simulink model "RPBSIDblocks"  (Simulink 7.4)
settings: Solver=ode45  StartTime=0.0  StopTime=10.0  RelTol=1e-3
undefined symbols (not defined in the file): Du, Dy, W
libraries: cstblocks x1
(part 1 of 2)
settings Model: Creator=ivohoutzager  LastModifiedBy=Ivo
settings OptimizationCC: InitFltsAndDblsToZero=on
settings DebuggingCC: SaveWithParameterizedLinksMsg=none  MultiTaskCondExecSysMsg=none
settings HardwareCC: TargetHWDeviceType=32-bit Generic
settings RTWCC: IncludeERTFirstTime=on
settings GRTTargetCC: TargetFcnLib=ansi_tfl_tmw.mat

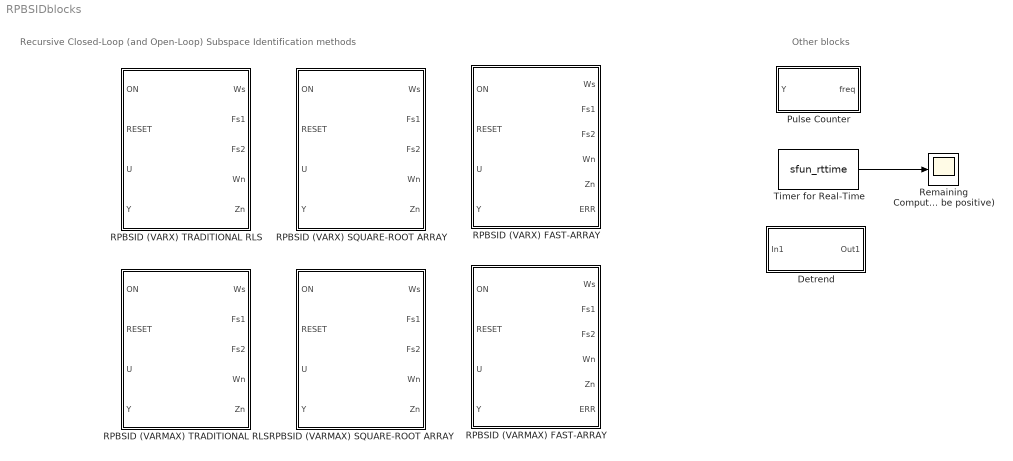
== system RPBSIDblocks ==
  note: Recursive Closed-Loop (and Open-Loop)
      | Subspace Identification methods
  note: Other blocks
  Detrend : Subsystem
  Pulse Counter : Stateflow chart
  RPBSID (VARMAX) FAST-ARRAY : Stateflow chart
  RPBSID (VARMAX) SQUARE-ROOT ARRAY : Stateflow chart
  RPBSID (VARMAX) TRADITIONAL RLS : Stateflow chart
  RPBSID (VARX) FAST-ARRAY : Stateflow chart
  RPBSID (VARX) SQUARE-ROOT ARRAY : Stateflow chart
  RPBSID (VARX) TRADITIONAL RLS : Stateflow chart
  Remaining Computation Time (must be positive) : Scope
      settings: TimeRange=10  YMin=-0.01  YMax=0.01
  Timer for Real-Time : S-Function  FunctionName=sfun_rttime  Parameters=1  EnableBusSupport=off
  wires:
  Timer for Real-Time/1 -> Remaining Computation Time (must be positive)/1

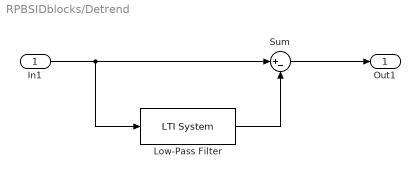
== system RPBSIDblocks/Detrend ==
  In1 : Inport  OutDataType=fixdt(1, 16)  OutScaling=2^0
  Low-Pass Filter : cstblocks/LTI System  SystemSampleTime=-1  sys=LP  IC=[]
  Sum : Sum  Inputs=|+-  OutDataType=fixdt(1, 16)  OutScaling=2^0
  Out1 : Outport  OutDataType=fixdt(1, 16)  OutScaling=2^0
  wires:
  In1/1 -> Low-Pass Filter/1, Sum/1
  Low-Pass Filter/1 -> Sum/2
  Sum/1 -> Out1/1

== matlab function RPBSID (VARMAX) SQUARE-ROOT ARRAY ==
  data: ON input double; RESET input double; Ws output double; Fs1 output double; Fs2 output double; U input double; Y input double size=2; Wn output double; Zn output double; W parameter double; Du parameter double; Dy parameter double
function [Ws,Fs1,Fs2,Wn,Zn] = rpbsid(ON,RESET,U,Y,W,Du,Dy)
%RPBSID Closed-loop recursive predictor-based subspace identification (VARX)

% Input definitions
% U input sample
% Y output sample
% W weight matrix (from workspace)
% Du input scaling matrix from sigscale (from workspace)
% Dy output scaling matric from sigscale (from workspace)

% Common paremeters
r = 1;         % number if inpuh
l = 2;         % number of outpuh
m = 2*l+r;
n = 7;         % number of states
h = 0.05;      % sample time

% Parameters for identification
p = 50;        % past window
f = 50;        % future window
noD = 0;       % no direct feedtrough
off = 1;       % remove offset in Markov estimation
weight = 0;    % apply transformation filter

% Parameters for adaptive filters
lambda1 = 0.999; % initial forgetting factor (~= 1 - 2/window)
lambda2 = 0.999; % initial forgetting factor (~= 1 - 2/window)
lambda3 = 0.999; % initial forgetting factor (~= 1 - 2/window)
ireg1 = 100;     % initial regularisation
ireg2 = 1e-6;    % initial regularisation
ireg3 = 1e-6;    % initial regularisation
reg1 = 1;        % initial regularisation

% Initialization
startA = 3;

% Initialize if needed
persistent Plk VARX LK Pcd Pabk ABK CD U1 Y1 X X1 E1 Zp w k start saw
if isempty(Plk) || RESET
    % Initialisation of Markov estimation problem
    if noD
        if off
            Plk = (1/sqrt(ireg1)).*eye(p*m+1);
            VARX = zeros(l,p*m+1);
        else
            Plk = (1/sqrt(ireg1)).*eye(p*m);
            VARX = zeros(l,p*m);
        end
    else
        if off
            Plk = (1/sqrt(ireg1)).*eye(p*m+r+1);
            VARX = zeros(l,p*m+r+1);
        else
            Plk = (1/sqrt(ireg1)).*eye(p*m+r);
            VARX = zeros(l,p*m+r);
        end
    end
    saw = 0;
    
    % Initialisation of the LambdaKappa
    LK = zeros(f*l,m*p);
    
    % Initialisation the estimate of ABK
    Pabk = (1/sqrt(ireg2)).*eye(n+r+l);
    ABK = [zeros(n) zeros(n,r) zeros(n,l)];
    
    if noD
        % Initialisation the estimate of CD
        Pcd = (1/sqrt(ireg3)).*eye(n);
        CD = zeros(l,n);
    else
        % Initialisation the estimate of CD and e
        Pcd = (1/sqrt(ireg3)).*eye(n+r);
        CD = [zeros(l,n) zeros(l,r)];
    end

    % Store vectors for next iteration
    Y1 = zeros(l,1);
    U1 = zeros(r,1);
    X1 = zeros(n,1);
    X = zeros(n,1);
    E1 = zeros(l,1);
    Zp = zeros(p*m,1); 
    
    % Frequency grid
    w = logspace(-1,1,300);
    k = 1;
    start = 1;
end

% Start RPBSID iff ON is set
if ON > 0.5
    
    % Scale input and output
    U = diag(1./diag(Du))*U;
    Y = diag(1./diag(Dy))*Y;
    
    % New signal vector
    Zp(1:(p-1)*m,1) = Zp(m+1:p*m,1);
    Zp((p-1)*m+1:p*m,1) = [U1; Y1; E1];
    if noD
        if off
            Z = [Zp; 1];
        else
            Z = Zp;
        end
    else
        if off
            Z = [Zp; U; 1];
        else
            Z = [Zp; U];
        end
    end

    if (start < 0.5) || (k >= p)
        % Solve Markov estimation problem recursively
        if reg1 ~= 0
            [VARX,Plk,saw] = inverseQRreg(Z,Y,VARX,Plk,lambda1,reg1,saw);
            E1 = Y - VARX*Z;
        else
            [VARX,Plk] = inverseQR(Z,Y,VARX,Plk,lambda1);
            E1 = Y - VARX*Z;
        end
    end
    
    if (start < 0.5) || (k >= startA*p)
        % Construction of LambdaKappa
        LK = zeros(f*l,p*m);
        if ~weight
            for i = 0:f-1
                for h = 0:p-i-1
                    LK(i*l+(1:l),(i+h)*m+(1:m)) = VARX(:,h*m+(1:m));
                end
            end
        else
            for i = 0:f-1
                for h = 0:p-i-1
                    LK(i*l+(1:l),(i+h)*m+(1:m)) = VARX(:,h*m+(1:m));
                end
                if i ~= 0
                    for j = 0:i-1
                        LK(i*l+(1:l),:) = LK(i*l+(1:l),:) + VARX(:,(p-i+j)*m+r+(1:l))*LK(j*l+(1:l),:);
                    end
                end
            end
        end
        
        % The estimation of the state vector
        X = W*LK*Zp;
    end
    
    if (start < 0.5) || (k >= startA*p+1)
        % The estimation of the system matrices
        if noD
            [CD,Pcd] = inverseQR(X1,Y1,CD,Pcd,lambda2);
            R1 = Y1-CD*X1;
        else
            [CD,Pcd] = inverseQR([X1; U1],Y1,CD,Pcd,lambda2);
            R1 = Y1-CD*[X1; U1];
        end
        [ABK,Pabk] = inverseQR([X1; U1; R1],X,ABK,Pabk,lambda3);
    end
        
    % Store vectors and matrices for next iteration
    if (start < 0.5) || (k >= startA*p)
        X1 = X;
    end
    Y1 = Y;
    U1 = U;
end

% Store state-space matrices
A = ABK(:,1:n);
B = ABK(:,n+1:n+r)*diag(1./diag(Du));
C = Dy*CD(:,1:n);
if noD
    D = zeros(l,r);
else
    D = Dy*CD(:,n+1:end)*diag(1./diag(Du));
end
K = ABK(:,n+r+1:n+r+l);

% Calculate damping and frequencies
[Wn,Zn] = damp(A,h);

% Calculate frequency response
Ws = w(k);
Fs = real(abs(C*((exp(sqrt(complex(-1))*h*Ws*2*pi).*eye(n) - A)\B)+D));
Ws = log10(Ws);
if Fs(1) < 1e-5
    Fs1 = -100;
else
    Fs1 = 20*log10(Fs(1));
end
if Fs(2) < 1e-5
    Fs2 = -100;
else
    Fs2 = 20*log10(Fs(2));
end

% Update counter
if k >= length(w)
    start = 0;
    k = 1;
else
    k = k+1;
end

end % END RPBSID


function [theta,P,saw,R] = inverseQRreg(z,y,theta,P,lambda,reg,saw)
%INVERSEQR Square-Root Recursive Least Squares update (inverse QR)
[mz,nz] = size(z);

% Do regularization update first
eta = zeros(mz,nz);
if saw > (mz-0.5)
   saw = 1;
else
   saw = saw + 1; 
end
eta(saw) = sqrt((1-lambda^mz)*reg);
etap = eta'*P;
M = [eye(nz) etap; zeros(mz,nz) P];
for i = (size(P,2)+nz):-1:2
    % determine Givens rotation parameters
    if M(1,i) == 0
    elseif M(1,1) == 0
        % swap
        h = M(:,i);
        M(:,i) = -M(:,1);
        M(:,1) = h;
    else
        % determine Givens rotation parameters
        rho = M(1,i)/M(1,1);
        c = sqrt(1+abs(rho)^2);
        
        % apply givens rotation using mixed-downdating (more numeric stable)
        M(:,1) = (M(:,1) + rho.*M(:,i))./c;
        M(:,i) = -rho.*M(:,1) + c.*M(:,i);
    end
end
P = M(nz+1:end,nz+1:end);

% Do data update
zp = z'*P;
M = [eye(nz) (zp)./sqrt(lambda); zeros(mz,nz) P./sqrt(lambda)];
for i = (size(P,2)+nz):-1:2
    % determine Givens rotation parameters
    if M(1,i) == 0
    elseif M(1,1) == 0
        % swap
        h = M(:,i);
        M(:,i) = -M(:,1);
        M(:,1) = h;
    else
        % determine Givens rotation parameters
        rho = M(1,i)/M(1,1);
        c = sqrt(1+abs(rho)^2);
        
        % apply givens rotation using mixed-downdating (more numeric stable)
        M(:,1) = (M(:,1) + rho.*M(:,i))./c;
        M(:,i) = -rho.*M(:,1) + c.*M(:,i);
    end
end
G = M(nz+1:end,1:nz)/M(1:nz,1:nz);
P = M(nz+1:end,nz+1:end);
E = y - theta*z;
theta = theta + E*G';
if nargout == 3
    R = norm(y - theta*z);
end
end

function [theta,P,R] = inverseQR(z,y,theta,P,lambda)
%INVERSEQR Square-Root Recursive Least Squares update (inverse QR)

[mz,nz] = size(z);
zp = z'*P;
M = [eye(nz) (zp)./sqrt(lambda); zeros(mz,nz) P./sqrt(lambda)];
for i = (size(P,2)+nz):-1:2
    % determine Givens rotation parameters
    if M(1,i) == 0
    elseif M(1,1) == 0
        % swap
        h = M(:,i);
        M(:,i) = -M(:,1);
        M(:,1) = h;
    else
        % determine Givens rotation parameters
        rho = M(1,i)/M(1,1);
        c = sqrt(1+abs(rho)^2);
        
        % apply givens rotation using mixed-downdating (more numeric stable)
        M(:,1) = (M(:,1) + rho.*M(:,i))./c;
        M(:,i) = -rho.*M(:,1) + c.*M(:,i);
    end
end
G = M(nz+1:end,1:nz)/M(1:nz,1:nz);
P = M(nz+1:end,nz+1:end);
E = y - theta*z;
theta = theta + E*G';
if nargout == 3
    R = norm(y - theta*z);
end
end


function [wn,z] = damp(a,h)
%DAMP  Natural frequency and damping

% Calculate eigenvalues
r = eig(a);
[~,I] = sort(real(r));
r = r(I);

% Discrete: compute equivalent S-plane poles
if any(r) == 0
    z = zeros(size(r));
    wn = zeros(size(r));
else
    s = log(r)/h;
    f = abs(s);
    wn = f;
    z = -real(s)./f;
end
end

%% UNCOMMENT THE LATTER FOR OLDER MATLAB VERSIONS

% function y = log10(x)
% %LOG10  Common (base 10) logarithm.
% y = log(x)/log(10);
% end

% function E = eig(A)
% % Compute eigenvalues of matrix
% tol = 1e-4;
% maxit = 20;
% n = size(A,1);
% C = complex(A,zeros(n));
% A1 = C(n,n);
% E = complex(zeros(n,1),zeros(n,1));
% I = eye(n);
% for k2 = n:-1:2
%     k = 1;
%     brk = 0;
%     while k <= maxit && brk <= 0.5
%         mu = qrshift(C(k2+(-1:0),k2+(-1:0)));
%         M = (C - mu(1).*I);
%         [Q,R] = qr(M);
%         C = (R*Q + mu(1).*I);
%         if abs(abs(A1)-abs(C(k2,k2))) < tol
%             brk = 1;
%             A1 = C(k2-1,k2-1);
%         else
%             A1 = C(k2,k2);
%         end
%         k = k+1;
%     end
%     E(k2) = C(k2,k2);
%     C(k2,1:n) = 0;
%     C(1:n,k2) = 0;
%     I(k2,k2) = 0;
% end
% E(1) = C(1,1);
% E = sort(E);
% end

% function mu = qrshift(A)
% % Compute the Wilkinson double shift
% 
% trA = A(1,1) + A(2,2);
% detA =  A(1,1)*A(2,2) - A(1,2)*A(2,1);
% 
% mu1 = 0.5*(trA + sqrt(trA^2-4*detA));
% mu2 = 0.5*(trA - sqrt(trA^2-4*detA));
% if abs(abs(A(2,2)) - abs(mu1)) < abs(abs(A(2,2)) - abs(mu2))
%     mu = mu1;
% else
%     mu = mu2;
% end
% end

== matlab function RPBSID (VARX) SQUARE-ROOT ARRAY ==
  data: ON input double; RESET input double; Ws output double; Fs1 output double; Fs2 output double; U input double; Y input double size=2; Wn output double; Zn output double; W parameter double; Du parameter double; Dy parameter double
function [Ws,Fs1,Fs2,Wn,Zn] = rpbsid(ON,RESET,U,Y,W,Du,Dy)
%RPBSID Closed-loop recursive predictor-based subspace identification (VARX)

% Input definitions
% U input sample
% Y output sample
% W weight matrix (from workspace)
% Du input scaling matrix from sigscale (from workspace)
% Dy output scaling matric from sigscale (from workspace)

% Common paremeters
r = 1;         % number if inpuh
l = 2;         % number of outpuh
m = l+r;
n = 7;         % number of states
h = 0.05;      % sample time

% Parameters for identification
p = 50;        % past window
f = 50;        % future window
noD = 0;       % no direct feedtrough
off = 1;       % remove offset in Markov estimation
weight = 0;    % apply transformation filter

% Parameters for adaptive filters
lambda1 = 0.999; % initial forgetting factor (~= 1 - 2/window)
lambda2 = 0.999; % initial forgetting factor (~= 1 - 2/window)
lambda3 = 0.999; % initial forgetting factor (~= 1 - 2/window)
ireg1 = 100;     % initial regularisation
ireg2 = 1e-6;    % initial regularisation
ireg3 = 1e-6;    % initial regularisation
reg1 = 1;        % initial regularisation

% Initialization
startA = 3;

% Initialize if needed
persistent Plk VARX LK Pcd Pabk ABK CD U1 Y1 X X1 Zp w k start saw
if isempty(Plk)
    % Initialisation of Markov estimation problem
    if noD
        if off
            Plk = (1/sqrt(ireg1)).*eye(p*m+1);
            VARX = zeros(l,p*m+1);
        else
            Plk = (1/sqrt(ireg1)).*eye(p*m);
            VARX = zeros(l,p*m);
        end
    else
        if off
            Plk = (1/sqrt(ireg1)).*eye(p*m+r+1);
            VARX = zeros(l,p*m+r+1);
        else
            Plk = (1/sqrt(ireg1)).*eye(p*m+r);
            VARX = zeros(l,p*m+r);
        end
    end
    saw = 0;
    
    % Initialisation of the LambdaKappa
    LK = zeros(f*l,m*p);
    
    % Initialisation the estimate of ABK
    Pabk = (1/sqrt(ireg2)).*eye(n+r+l);
    ABK = [zeros(n) zeros(n,r) zeros(n,l)];
    
    if noD
        % Initialisation the estimate of CD
        Pcd = (1/sqrt(ireg3)).*eye(n);
        CD = zeros(l,n);
    else
        % Initialisation the estimate of CD and e
        Pcd = (1/sqrt(ireg3)).*eye(n+r);
        CD = [zeros(l,n) zeros(l,r)];
    end

    % Store vectors for next iteration
    Y1 = zeros(l,1);
    U1 = zeros(r,1);
    X1 = zeros(n,1);
    X = zeros(n,1);
    Zp = zeros(p*m,1); 
    
    % Frequency grid
    w = logspace(-1,1,300);
    k = 1;
    start = 1;
end

% Start RPBSID iff ON is set
if ON > 0.5
    
    % Scale input and output
    U = diag(1./diag(Du))*U;
    Y = diag(1./diag(Dy))*Y;
    
    % New signal vector
    Zp(1:(p-1)*m,1) = Zp(m+1:p*m,1);
    Zp((p-1)*m+1:p*m,1) = [U1; Y1];
    if noD
        if off
            Z = [Zp; 1];
        else
            Z = Zp;
        end
    else
        if off
            Z = [Zp; U; 1];
        else
            Z = [Zp; U];
        end
    end

    if (start < 0.5) || (k >= p)
        % Solve Markov estimation problem recursively
        if reg1 ~= 0
            [VARX,Plk,saw] = inverseQRreg(Z,Y,VARX,Plk,lambda1,reg1,saw);
        else
            [VARX,Plk] = inverseQR(Z,Y,VARX,Plk,lambda1);
        end
    end
    
    if (start < 0.5) || (k >= startA*p)
        % Construction of LambdaKappa
        LK = zeros(f*l,p*m);
        if ~weight
            for i = 0:f-1
                for h = 0:p-i-1
                    LK(i*l+(1:l),(i+h)*m+(1:m)) = VARX(:,h*m+(1:m));
                end
            end
        else
            for i = 0:f-1
                for h = 0:p-i-1
                    LK(i*l+(1:l),(i+h)*m+(1:m)) = VARX(:,h*m+(1:m));
                end
                if i ~= 0
                    for j = 0:i-1
                        LK(i*l+(1:l),:) = LK(i*l+(1:l),:) + VARX(:,(p-i+j)*m+r+(1:l))*LK(j*l+(1:l),:);
                    end
                end
            end
        end
        
        % The estimation of the state vector
        X = W*LK*Zp;
    end
    
    if (start < 0.5) || (k >= startA*p+1)
        % The estimation of the system matrices
        if noD
            [CD,Pcd] = inverseQR(X1,Y1,CD,Pcd,lambda2);
            R1 = Y1-CD*X1;
        else
            [CD,Pcd] = inverseQR([X1; U1],Y1,CD,Pcd,lambda2);
            R1 = Y1-CD*[X1; U1];
        end
        [ABK,Pabk] = inverseQR([X1; U1; R1],X,ABK,Pabk,lambda3);
    end
        
    % Store vectors and matrices for next iteration
    if (start < 0.5) || (k >= startA*p)
        X1 = X;
    end
    Y1 = Y;
    U1 = U;
end

% Store state-space matrices
A = ABK(:,1:n);
B = ABK(:,n+1:n+r)*diag(1./diag(Du));
C = Dy*CD(:,1:n);
if noD
    D = zeros(l,r);
else
    D = Dy*CD(:,n+1:end)*diag(1./diag(Du));
end
K = ABK(:,n+r+1:n+r+l);

% Calculate damping and frequencies
[Wn,Zn] = damp(A,h);

% Calculate frequency response
Ws = w(k);
Fs = real(abs(C*((exp(sqrt(complex(-1))*h*Ws*2*pi).*eye(n) - A)\B)+D));
Ws = log10(Ws);
if Fs(1) < 1e-5
    Fs1 = -100;
else
    Fs1 = 20*log10(Fs(1));
end
if Fs(2) < 1e-5
    Fs2 = -100;
else
    Fs2 = 20*log10(Fs(2));
end

% Update counter
if k >= length(w)
    start = 0;
    k = 1;
else
    k = k+1;
end

end % END RPBSID


function [theta,P,saw,R] = inverseQRreg(z,y,theta,P,lambda,reg,saw)
%INVERSEQR Square-Root Recursive Least Squares update (inverse QR)
[mz,nz] = size(z);

% Do regularization update first
eta = zeros(mz,nz);
if saw > (mz-0.5)
   saw = 1;
else
   saw = saw + 1; 
end
eta(saw) = sqrt((1-lambda^mz)*reg);
M = [eye(nz) eta'*P; zeros(mz,nz) P];
for i = (size(P,2)+nz):-1:2
    % determine Givens rotation parameters
    if M(1,i) == 0
    elseif M(1,1) == 0
        % swap
        h = M(:,i);
        M(:,i) = -M(:,1);
        M(:,1) = h;
    else
        % determine Givens rotation parameters
        rho = M(1,i)/M(1,1);
        c = sqrt(1+abs(rho)^2);
        
        % apply givens rotation using mixed-downdating (more numeric stable)
        M(:,1) = (M(:,1) + rho.*M(:,i))./c;
        M(:,i) = -rho.*M(:,1) + c.*M(:,i);
    end
end
P = M(nz+1:end,nz+1:end);

% Do data update
zp = z'*P;
M = [eye(nz) (zp)./sqrt(lambda); zeros(mz,nz) P./sqrt(lambda)];
for i = (size(P,2)+nz):-1:2
    % determine Givens rotation parameters
    if M(1,i) == 0
    elseif M(1,1) == 0
        % swap
        h = M(:,i);
        M(:,i) = -M(:,1);
        M(:,1) = h;
    else
        % determine Givens rotation parameters
        rho = M(1,i)/M(1,1);
        c = sqrt(1+abs(rho)^2);
        
        % apply givens rotation using mixed-downdating (more numeric stable)
        M(:,1) = (M(:,1) + rho.*M(:,i))./c;
        M(:,i) = -rho.*M(:,1) + c.*M(:,i);
    end
end
G = M(nz+1:end,1:nz)/M(1:nz,1:nz);
P = M(nz+1:end,nz+1:end);
E = y - theta*z;
theta = theta + E*G';
if nargout == 3
    R = norm(y - theta*z);
end
end

function [theta,P,R] = inverseQR(z,y,theta,P,lambda)
%INVERSEQR Square-Root Recursive Least Squares update (inverse QR)

[mz,nz] = size(z);
zp = z'*P;
M = [eye(nz) (zp)./sqrt(lambda); zeros(mz,nz) P./sqrt(lambda)];
for i = (size(P,2)+nz):-1:2
    % determine Givens rotation parameters
    if M(1,i) == 0
    elseif M(1,1) == 0
        % swap
        h = M(:,i);
        M(:,i) = -M(:,1);
        M(:,1) = h;
    else
        % determine Givens rotation parameters
        rho = M(1,i)/M(1,1);
        c = sqrt(1+abs(rho)^2);
        
        % apply givens rotation using mixed-downdating (more numeric stable)
        M(:,1) = (M(:,1) + rho.*M(:,i))./c;
        M(:,i) = -rho.*M(:,1) + c.*M(:,i);
    end
end
G = M(nz+1:end,1:nz)/M(1:nz,1:nz);
P = M(nz+1:end,nz+1:end);
E = y - theta*z;
theta = theta + E*G';
if nargout == 3
    R = norm(y - theta*z);
end
end


function [wn,z] = damp(a,h)
%DAMP  Natural frequency and damping

% Calculate eigenvalues
r = eig(a);
[~,I] = sort(real(r));
r = r(I);

% Discrete: compute equivalent S-plane poles
if any(r) == 0
    z = zeros(size(r));
    wn = zeros(size(r));
else
    s = log(r)/h;
    f = abs(s);
    wn = f;
    z = -real(s)./f;
end
end

%% UNCOMMENT THE LATTER FOR OLDER MATLAB VERSIONS

% function y = log10(x)
% %LOG10  Common (base 10) logarithm.
% y = log(x)/log(10);
% end

% function E = eig(A)
% % Compute eigenvalues of matrix
% tol = 1e-4;
% maxit = 20;
% n = size(A,1);
% C = complex(A,zeros(n));
% A1 = C(n,n);
% E = complex(zeros(n,1),zeros(n,1));
% I = eye(n);
% for k2 = n:-1:2
%     k = 1;
%     brk = 0;
%     while k <= maxit && brk <= 0.5
%         mu = qrshift(C(k2+(-1:0),k2+(-1:0)));
%         M = (C - mu(1).*I);
%         [Q,R] = qr(M);
%         C = (R*Q + mu(1).*I);
%         if abs(abs(A1)-abs(C(k2,k2))) < tol
%             brk = 1;
%             A1 = C(k2-1,k2-1);
%         else
%             A1 = C(k2,k2);
%         end
%         k = k+1;
%     end
%     E(k2) = C(k2,k2);
%     C(k2,1:n) = 0;
%     C(1:n,k2) = 0;
%     I(k2,k2) = 0;
% end
% E(1) = C(1,1);
% E = sort(E);
% end

% function mu = qrshift(A)
% % Compute the Wilkinson double shift
% 
% trA = A(1,1) + A(2,2);
% detA =  A(1,1)*A(2,2) - A(1,2)*A(2,1);
% 
% mu1 = 0.5*(trA + sqrt(trA^2-4*detA));
% mu2 = 0.5*(trA - sqrt(trA^2-4*detA));
% if abs(abs(A(2,2)) - abs(mu1)) < abs(abs(A(2,2)) - abs(mu2))
%     mu = mu1;
% else
%     mu = mu2;
% end
% end

== matlab function RPBSID (VARX) TRADITIONAL RLS ==
  data: ON input double; RESET input double; Ws output double; Fs1 output double; Fs2 output double; U input double; Y input double size=2; Wn output double; Zn output double; W parameter double; Du parameter double; Dy parameter double
function [Ws,Fs1,Fs2,Wn,Zn] = rpbsid(ON,RESET,U,Y,W,Du,Dy)
%RPBSID Closed-loop recursive predictor-based subspace identification (VARX)

% Input definitions
% U input sample
% Y output sample
% W weight matrix (from workspace)
% Du input scaling matrix from sigscale (from workspace)
% Dy output scaling matric from sigscale (from workspace)

% Common paremeters
r = 1;         % number if inpuh
l = 2;         % number of outpuh
m = l+r;
n = 7;         % number of states
h = 0.05;      % sample time

% Parameters for identification
p = 50;        % past window
f = 50;        % future window
noD = 0;       % no direct feedtrough
off = 1;       % remove offset in Markov estimation
weight = 0;    % apply transformation filter

% Parameters for adaptive filters
lambda1 = 0.999; % initial forgetting factor (~= 1 - 2/window)
lambda2 = 0.999; % initial forgetting factor (~= 1 - 2/window)
lambda3 = 0.999; % initial forgetting factor (~= 1 - 2/window)
ireg1 = 100;     % initial regularisation
ireg2 = 1e-6;    % initial regularisation
ireg3 = 1e-6;    % initial regularisation
reg1 = 1;        % initial regularisation

% Initialization
startA = 3;

% Initialize if needed
persistent Plk VARX LK Pcd Pabk ABK CD U1 Y1 X X1 Zp w k start saw
if isempty(Plk)
    % Initialisation of Markov estimation problem
    if noD
        if off
            Plk = (1/ireg1).*eye(p*m+1);
            VARX = zeros(l,p*m+1);
        else
            Plk = (1/ireg1).*eye(p*m);
            VARX = zeros(l,p*m);
        end
    else
        if off
            Plk = (1/ireg1).*eye(p*m+r+1);
            VARX = zeros(l,p*m+r+1);
        else
            Plk = (1/ireg1).*eye(p*m+r);
            VARX = zeros(l,p*m+r);
        end
    end
    saw = 0;
    
    % Initialisation of the LambdaKappa
    LK = zeros(f*l,m*p);
    
    % Initialisation the estimate of ABK
    Pabk = (1/ireg2).*eye(n+r+l);
    ABK = [zeros(n) zeros(n,r) zeros(n,l)];
    
    if noD
        % Initialisation the estimate of CD
        Pcd = (1/ireg3).*eye(n);
        CD = zeros(l,n);
    else
        % Initialisation the estimate of CD and e
        Pcd = (1/ireg3).*eye(n+r);
        CD = [zeros(l,n) zeros(l,r)];
    end

    % Store vectors for next iteration
    Y1 = zeros(l,1);
    U1 = zeros(r,1);
    X1 = zeros(n,1);
    X = zeros(n,1);
    Zp = zeros(p*m,1); 
    
    % Frequency grid
    w = logspace(-1,1,300);
    k = 1;
    start = 1;
end

% Start RPBSID iff ON is set
if ON > 0.5
    
    % Scale input and output
    U = diag(1./diag(Du))*U;
    Y = diag(1./diag(Dy))*Y;
    
    % New signal vector
    Zp(1:(p-1)*m,1) = Zp(m+1:p*m,1);
    Zp((p-1)*m+1:p*m,1) = [U1; Y1];
    if noD
        if off
            Z = [Zp; 1];
        else
            Z = Zp;
        end
    else
        if off
            Z = [Zp; U; 1];
        else
            Z = [Zp; U];
        end
    end

    if (start < 0.5) || (k >= p)
        % Solve Markov estimation problem recursively
        if reg1 ~= 0
            [VARX,Plk,saw] = rls_ew_reg(Z,Y,VARX,Plk,lambda1,reg1,saw);
        else
            [VARX,Plk] = rls_ew(Z,Y,VARX,Plk,lambda1);
        end
    end
    
    if (start < 0.5) || (k >= startA*p)
        % Construction of LambdaKappa
        LK = zeros(f*l,p*m);
        if ~weight
            for i = 0:f-1
                for h = 0:p-i-1
                    LK(i*l+(1:l),(i+h)*m+(1:m)) = VARX(:,h*m+(1:m));
                end
            end
        else
            for i = 0:f-1
                for h = 0:p-i-1
                    LK(i*l+(1:l),(i+h)*m+(1:m)) = VARX(:,h*m+(1:m));
                end
                if i ~= 0
                    for j = 0:i-1
                        LK(i*l+(1:l),:) = LK(i*l+(1:l),:) + VARX(:,(p-i+j)*m+r+(1:l))*LK(j*l+(1:l),:);
                    end
                end
            end
        end
        
        % The estimation of the state vector
        X = W*LK*Zp;
    end
    
    if (start < 0.5) || (k >= startA*p+1)
        % The estimation of the system matrices
        if noD
            [CD,Pcd] = rls_ew(X1,Y1,CD,Pcd,lambda2);
            R1 = Y1-CD*X1;
        else
            [CD,Pcd] = rls_ew([X1; U1],Y1,CD,Pcd,lambda2);
            R1 = Y1-CD*[X1; U1];
        end
        [ABK,Pabk] = rls_ew([X1; U1; R1],X,ABK,Pabk,lambda3);
    end
        
    % Store vectors and matrices for next iteration
    if (start < 0.5) || (k >= startA*p)
        X1 = X;
    end
    Y1 = Y;
    U1 = U;
end

% Store state-space matrices
A = ABK(:,1:n);
B = ABK(:,n+1:n+r)*diag(1./diag(Du));
C = Dy*CD(:,1:n);
if noD
    D = zeros(l,r);
else
    D = Dy*CD(:,n+1:end)*diag(1./diag(Du));
end
K = ABK(:,n+r+1:n+r+l);

% Calculate damping and frequencies
[Wn,Zn] = damp(A,h);

% Calculate frequency response
Ws = w(k);
Fs = real(abs(C*((exp(sqrt(complex(-1))*h*Ws*2*pi).*eye(n) - A)\B)+D));
Ws = log10(Ws);
if Fs(1) < 1e-5
    Fs1 = -100;
else
    Fs1 = 20*log10(Fs(1));
end
if Fs(2) < 1e-5
    Fs2 = -100;
else
    Fs2 = 20*log10(Fs(2));
end

% Update counter
if k >= length(w)
    start = 0;
    k = 1;
else
    k = k+1;
end

end % END RPBSID


function [theta,P,saw,R] = rls_ew_reg(z,y,theta,P,lambda,reg,saw)
%RLS_EW Exponentially Weighted RLS iteration
%  [THETA,P,R]=RLS_EW(Z,Y,THETA,P,LAMBDA) applies one iteration of
%  exponentially weighted regularized least-squares problem. In recursive
%  least-squares, we deal with the issue of an inceasing amount of date Z
%  and Y. At each iteration, THETA is the solution. The scalar LAMBDA is
%  called the forgetting factor since past data are exponentially weighted
%  less heavily than more recent data.

%  Ivo Houtzager
%  Delft Center of Systems and Control
%  The Netherlands, 2010

% Do regularization update first
[mz,nz] = size(z);
eta = zeros(mz,nz);
if saw > (mz-0.5)
   saw = 1;
else
   saw = saw + 1; 
end
eta(saw) = sqrt((1-lambda^mz)*reg);
P = (P - P*(eta*eta')*P./(1 + eta'*P*eta));

% Exponentially-Weighted, Tracking, Regularized, Least-Squares Iteration
P = (1/lambda).*(P - P*(z*z')*P./(lambda + z'*P*z));
P = 0.5.*(P+P'); % force symmetric
e = y - theta*z;
theta = theta + e*z'*P;

if nargout == 3
    R = norm(y - theta*z);
end
end % end of function RLS_EW

function [theta,P,R] = rls_ew(z,y,theta,P,lambda)
%RLS_EW Exponentially Weighted RLS iteration
%  [THETA,P,R]=RLS_EW(Z,Y,THETA,P,LAMBDA) applies one iteration of
%  exponentially weighted regularized least-squares problem. In recursive
%  least-squares, we deal with the issue of an inceasing amount of date Z
%  and Y. At each iteration, THETA is the solution. The scalar LAMBDA is
%  called the forgetting factor since past data are exponentially weighted
%  less heavily than more recent data.

%  Ivo Houtzager
%  Delft Center of Systems and Control
%  The Netherlands, 2010

% Exponentially-Weighted, Tracking, Regularized, Least-Squares Iteration
P = (1/lambda).*(P - P*(z*z')*P./(lambda + z'*P*z));
P = 0.5.*(P+P'); % force symmetric
e = y - theta*z;
theta = theta + e*z'*P;
if nargout == 3
    R = norm(y - theta*z);
end
end % end of function RLS_EW


function [wn,z] = damp(a,h)
%DAMP  Natural frequency and damping

% Calculate eigenvalues
r = eig(a);
[~,I] = sort(real(r));
r = r(I);

% Discrete: compute equivalent S-plane poles
if any(r) == 0
    z = zeros(size(r));
    wn = zeros(size(r));
else
    s = log(r)/h;
    f = abs(s);
    wn = f;
    z = -real(s)./f;
end
end

%% UNCOMMENT THE LATTER FOR OLDER MATLAB VERSIONS

% function y = log10(x)
% %LOG10  Common (base 10) logarithm.
% y = log(x)/log(10);
% end

% function E = eig(A)
% % Compute eigenvalues of matrix
% tol = 1e-4;
% maxit = 20;
% n = size(A,1);
% C = complex(A,zeros(n));
% A1 = C(n,n);
% E = complex(zeros(n,1),zeros(n,1));
% I = eye(n);
% for k2 = n:-1:2
%     k = 1;
%     brk = 0;
%     while k <= maxit && brk <= 0.5
%         mu = qrshift(C(k2+(-1:0),k2+(-1:0)));
%         M = (C - mu(1).*I);
%         [Q,R] = qr(M);
%         C = (R*Q + mu(1).*I);
%         if abs(abs(A1)-abs(C(k2,k2))) < tol
%             brk = 1;
%             A1 = C(k2-1,k2-1);
%         else
%             A1 = C(k2,k2);
%         end
%         k = k+1;
%     end
%     E(k2) = C(k2,k2);
%     C(k2,1:n) = 0;
%     C(1:n,k2) = 0;
%     I(k2,k2) = 0;
% end
% E(1) = C(1,1);
% E = sort(E);
% end

% function mu = qrshift(A)
% % Compute the Wilkinson double shift
% 
% trA = A(1,1) + A(2,2);
% detA =  A(1,1)*A(2,2) - A(1,2)*A(2,1);
% 
% mu1 = 0.5*(trA + sqrt(trA^2-4*detA));
% mu2 = 0.5*(trA - sqrt(trA^2-4*detA));
% if abs(abs(A(2,2)) - abs(mu1)) < abs(abs(A(2,2)) - abs(mu2))
%     mu = mu1;
% else
%     mu = mu2;
% end
% end

== matlab function RPBSID (VARMAX) TRADITIONAL RLS ==
  data: ON input double; RESET input double; Ws output double; Fs1 output double; Fs2 output double; U input double; Y input double size=2; Wn output double; Zn output double; W parameter double; Du parameter double; Dy parameter double
function [Ws,Fs1,Fs2,Wn,Zn] = rpbsid(ON,RESET,U,Y,W,Du,Dy)
%RPBSID Closed-loop recursive predictor-based subspace identification (VARX)

% Input definitions
% U input sample
% Y output sample
% W weight matrix (from workspace)
% Du input scaling matrix from sigscale (from workspace)
% Dy output scaling matric from sigscale (from workspace)

% Common paremeters
r = 1;         % number if inpuh
l = 2;         % number of outpuh
m = 2*l+r;
n = 7;         % number of states
h = 0.05;      % sample time

% Parameters for identification
p = 50;        % past window
f = 50;        % future window
noD = 0;       % no direct feedtrough
off = 1;       % remove offset in Markov estimation
weight = 0;    % apply transformation filter

% Parameters for adaptive filters
lambda1 = 0.999; % initial forgetting factor (~= 1 - 2/window)
lambda2 = 0.999; % initial forgetting factor (~= 1 - 2/window)
lambda3 = 0.999; % initial forgetting factor (~= 1 - 2/window)
ireg1 = 100;     % initial regularisation
ireg2 = 1e-6;    % initial regularisation
ireg3 = 1e-6;    % initial regularisation
reg1 = 1;        % initial regularisation

% Initialization
startA = 3;

% Initialize if needed
persistent Plk VARX LK Pcd Pabk ABK CD U1 Y1 X X1 E1 Zp w k start saw
if isempty(Plk) || RESET
    % Initialisation of Markov estimation problem
    if noD
        if off
            Plk = (1/ireg1).*eye(p*m+1);
            VARX = zeros(l,p*m+1);
        else
            Plk = (1/ireg1).*eye(p*m);
            VARX = zeros(l,p*m);
        end
    else
        if off
            Plk = (1/ireg1).*eye(p*m+r+1);
            VARX = zeros(l,p*m+r+1);
        else
            Plk = (1/ireg1).*eye(p*m+r);
            VARX = zeros(l,p*m+r);
        end
    end
    saw = 0;
    
    % Initialisation of the LambdaKappa
    LK = zeros(f*l,m*p);
    
    % Initialisation the estimate of ABK
    Pabk = (1/ireg2).*eye(n+r+l);
    ABK = [zeros(n) zeros(n,r) zeros(n,l)];
    
    if noD
        % Initialisation the estimate of CD
        Pcd = (1/ireg3).*eye(n);
        CD = zeros(l,n);
    else
        % Initialisation the estimate of CD and e
        Pcd = (1/ireg3).*eye(n+r);
        CD = [zeros(l,n) zeros(l,r)];
    end

    % Store vectors for next iteration
    Y1 = zeros(l,1);
    U1 = zeros(r,1);
    X1 = zeros(n,1);
    X = zeros(n,1);
    E1 = zeros(l,1);
    Zp = zeros(p*m,1); 
    
    % Frequency grid
    w = logspace(-1,1,300);
    k = 1;
    start = 1;
end

% Start RPBSID iff ON is set
if ON > 0.5
    
    % Scale input and output
    U = diag(1./diag(Du))*U;
    Y = diag(1./diag(Dy))*Y;
    
    % New signal vector
    Zp(1:(p-1)*m,1) = Zp(m+1:p*m,1);
    Zp((p-1)*m+1:p*m,1) = [U1; Y1; E1];
    if noD
        if off
            Z = [Zp; 1];
        else
            Z = Zp;
        end
    else
        if off
            Z = [Zp; U; 1];
        else
            Z = [Zp; U];
        end
    end

    if (start < 0.5) || (k >= p)
        % Solve Markov estimation problem recursively
        if reg1 ~= 0
            [VARX,Plk,saw] = rls_ew_reg(Z,Y,VARX,Plk,lambda1,reg1,saw);
            E1 = Y - VARX*Z;
        else
            [VARX,Plk] = rls_ew_reg(Z,Y,VARX,Plk,lambda1);
            E1 = Y - VARX*Z;
        end
    end
    
    if (start < 0.5) || (k >= startA*p)
        % Construction of LambdaKappa
        LK = zeros(f*l,p*m);
        if ~weight
            for i = 0:f-1
                for h = 0:p-i-1
                    LK(i*l+(1:l),(i+h)*m+(1:m)) = VARX(:,h*m+(1:m));
                end
            end
        else
            for i = 0:f-1
                for h = 0:p-i-1
                    LK(i*l+(1:l),(i+h)*m+(1:m)) = VARX(:,h*m+(1:m));
                end
                if i ~= 0
                    for j = 0:i-1
                        LK(i*l+(1:l),:) = LK(i*l+(1:l),:) + VARX(:,(p-i+j)*m+r+(1:l))*LK(j*l+(1:l),:);
                    end
                end
            end
        end
        
        % The estimation of the state vector
        X = W*LK*Zp;
    end
    
    if (start < 0.5) || (k >= startA*p+1)
        % The estimation of the system matrices
        if noD
            [CD,Pcd] = rls_ew(X1,Y1,CD,Pcd,lambda2);
            R1 = Y1-CD*X1;
        else
            [CD,Pcd] = rls_ew([X1; U1],Y1,CD,Pcd,lambda2);
            R1 = Y1-CD*[X1; U1];
        end
        [ABK,Pabk] = rls_ew([X1; U1; R1],X,ABK,Pabk,lambda3);
    end
        
    % Store vectors and matrices for next iteration
    if (start < 0.5) || (k >= startA*p)
        X1 = X;
    end
    Y1 = Y;
    U1 = U;
end

% Store state-space matrices
A = ABK(:,1:n);
B = ABK(:,n+1:n+r)*diag(1./diag(Du));
C = Dy*CD(:,1:n);
if noD
    D = zeros(l,r);
else
    D = Dy*CD(:,n+1:end)*diag(1./diag(Du));
end
K = ABK(:,n+r+1:n+r+l);

% Calculate damping and frequencies
[Wn,Zn] = damp(A,h);

% Calculate frequency response
Ws = w(k);
Fs = real(abs(C*((exp(sqrt(complex(-1))*h*Ws*2*pi).*eye(n) - A)\B)+D));
Ws = log10(Ws);
if Fs(1) < 1e-5
    Fs1 = -100;
else
    Fs1 = 20*log10(Fs(1));
end
if Fs(2) < 1e-5
    Fs2 = -100;
else
    Fs2 = 20*log10(Fs(2));
end

% Update counter
if k >= length(w)
    start = 0;
    k = 1;
else
    k = k+1;
end

end % END RPBSID


function [theta,P,saw,R] = rls_ew_reg(z,y,theta,P,lambda,reg,saw)
%RLS_EW Exponentially Weighted RLS iteration
%  [THETA,P,R]=RLS_EW(Z,Y,THETA,P,LAMBDA) applies one iteration of
%  exponentially weighted regularized least-squares problem. In recursive
%  least-squares, we deal with the issue of an inceasing amount of date Z
%  and Y. At each iteration, THETA is the solution. The scalar LAMBDA is
%  called the forgetting factor since past data are exponentially weighted
%  less heavily than more recent data.

%  Ivo Houtzager
%  Delft Center of Systems and Control
%  The Netherlands, 2010

% Do regularization update first
[mz,nz] = size(z);
eta = zeros(mz,nz);
if saw > (mz-0.5)
   saw = 1;
else
   saw = saw + 1; 
end
eta(saw) = sqrt((1-lambda^mz)*reg);
P = (P - P*(eta*eta')*P./(1 + eta'*P*eta));

% Exponentially-Weighted, Tracking, Regularized, Least-Squares Iteration
P = (1/lambda).*(P - P*(z*z')*P./(lambda + z'*P*z));
P = 0.5.*(P+P'); % force symmetric
e = y - theta*z;
theta = theta + e*z'*P;

if nargout == 3
    R = norm(y - theta*z);
end
end % end of function RLS_EW

function [theta,P,R] = rls_ew(z,y,theta,P,lambda)
%RLS_EW Exponentially Weighted RLS iteration
%  [THETA,P,R]=RLS_EW(Z,Y,THETA,P,LAMBDA) applies one iteration of
%  exponentially weighted regularized least-squares problem. In recursive
%  least-squares, we deal with the issue of an inceasing amount of date Z
%  and Y. At each iteration, THETA is the solution. The scalar LAMBDA is
%  called the forgetting factor since past data are exponentially weighted
%  less heavily than more recent data.

%  Ivo Houtzager
%  Delft Center of Systems and Control
%  The Netherlands, 2010

% Exponentially-Weighted, Tracking, Regularized, Least-Squares Iteration
P = (1/lambda).*(P - P*(z*z')*P./(lambda + z'*P*z));
P = 0.5.*(P+P'); % force symmetric
e = y - theta*z;
theta = theta + e*z'*P;
if nargout == 3
    R = norm(y - theta*z);
end
end % end of function RLS_EW


function [wn,z] = damp(a,h)
%DAMP  Natural frequency and damping

% Calculate eigenvalues
r = eig(a);
[~,I] = sort(real(r));
r = r(I);

% Discrete: compute equivalent S-plane poles
if any(r) == 0
    z = zeros(size(r));
    wn = zeros(size(r));
else
    s = log(r)/h;
    f = abs(s);
    wn = f;
    z = -real(s)./f;
end
end

%% UNCOMMENT THE LATTER FOR OLDER MATLAB VERSIONS

% function y = log10(x)
% %LOG10  Common (base 10) logarithm.
% y = log(x)/log(10);
% end

% function E = eig(A)
% % Compute eigenvalues of matrix
% tol = 1e-4;
% maxit = 20;
% n = size(A,1);
% C = complex(A,zeros(n));
% A1 = C(n,n);
% E = complex(zeros(n,1),zeros(n,1));
% I = eye(n);
% for k2 = n:-1:2
%     k = 1;
%     brk = 0;
%     while k <= maxit && brk <= 0.5
%         mu = qrshift(C(k2+(-1:0),k2+(-1:0)));
%         M = (C - mu(1).*I);
%         [Q,R] = qr(M);
%         C = (R*Q + mu(1).*I);
%         if abs(abs(A1)-abs(C(k2,k2))) < tol
%             brk = 1;
%             A1 = C(k2-1,k2-1);
%         else
%             A1 = C(k2,k2);
%         end
%         k = k+1;
%     end
%     E(k2) = C(k2,k2);
%     C(k2,1:n) = 0;
%     C(1:n,k2) = 0;
%     I(k2,k2) = 0;
% end
% E(1) = C(1,1);
% E = sort(E);
% end

% function mu = qrshift(A)
% % Compute the Wilkinson double shift
% 
% trA = A(1,1) + A(2,2);
% detA =  A(1,1)*A(2,2) - A(1,2)*A(2,1);
% 
% mu1 = 0.5*(trA + sqrt(trA^2-4*detA));
% mu2 = 0.5*(trA - sqrt(trA^2-4*detA));
% if abs(abs(A(2,2)) - abs(mu1)) < abs(abs(A(2,2)) - abs(mu2))
%     mu = mu1;
% else
%     mu = mu2;
% end
% end
